simulink model "HW1_9723052"  (R2020b)
settings: Solver=VariableStepAuto  StartTime=0.0  StopTime=45  RelTol=1e-3
InitFcn:
  | run('Transmitter.m')
StopFcn:
  | RxStream = out.RxStream
  | run('Receiver.m')
  | MY = out.MY
values from neighbouring files (symbols this model uses):
  alpha = 0.2    [Transmitter.m]
  Frame = reshape(Frames.',[1,R_a*C_a])    [Transmitter.m]
  H = [ 0,1,1,1,0,1,0,0,1,1,1,0,1,1,0,0,1,1,0,0,0,0,1,1,1,0,0,1,1,1,0,1,1,0,0,0,1,1,0,1,0,       1,0,0,1,0,0,0,0,1,1,0,0,1,1,0,0,0,0,0,1,0,1,0,0,1,1,1,0,0,0,0,1,1,0,1,1,0,1,1,1,1,       1,1,1,1,0,0,1,0,1,0,0,0,0,0,0,0,1,0,0,0,1,1,0,1,1,1,0,1,1,1,0,1,0,1,0,1,0,0,1,1,1,       0,1,0,1,0 ]    [Transmitter.m]
  hd = h(2:end).*conj(h(1:end-1))    [Transmitter.m]
  M = 16    [Transmitter.m]
  Rs = 10e3    (= 10000)    [Transmitter.m]
  span = 20    [Transmitter.m]
  SPS = 8    [Transmitter.m]
undefined symbols (not defined in the file or in its folder): magnitude, pskmod
libraries: simulink x6, commdigbbndpm3 x5, commdigbbndam3 x4, dspstat3 x2, commfilt2 x2, commchan3 x1, dspsrcs4 x1
settings Model: Creator=win_10  LastModifiedBy=bpc

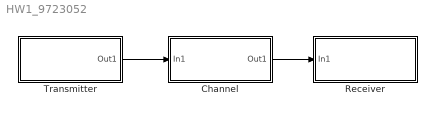
== system HW1_9723052 ==
  Channel : Subsystem
  Receiver : Subsystem
  Transmitter : Subsystem
  wires:
  Transmitter/1(Out1) -> Channel/1(In1)
  Channel/1(Out1) -> Receiver/1(In1)

== system HW1_9723052/Channel ==
  In1 : Inport
  AWGN Channel : commchan3/AWGN Channel  Commented=through  InputProcessing=Columns as channels (frame based)  seed=67  noiseMode="Signal to noise ratio  (Es/No)"  EbNodB=50  EsNodB=15  SNRdB=10  bitsPerSym=log2(M)  Ps=1/SPS  Tsym=1/Rs  variance=1
  Gain : Gain
  Out1 : Outport
  wires:
  In1/1 -> AWGN Channel/1
  AWGN Channel/1 -> Gain/1
  Gain/1 -> Out1/1

== system HW1_9723052/Receiver ==
  In1 : Inport
  Data Aided : Subsystem
  Downsample : DownSample  N=SPS  RateOptions=Allow multirate processing
  M&M : Subsystem  Commented=through
  Raised Cosine Receive Filter : commfilt2/Raised Cosine Receive Filter  filtType=Square root  R=alpha  filtSpan=span  N=SPS  downFactor=1  downOffset=0  filterGain=1  InputProcessing=Columns as channels (frame based)  RateOptions=Allow multirate processing  framing=Mute  checkCoeff=off  variableName=rcRxFilt  currentFiltSpan=span  D=(span)/2  inputOffset=0  sampMode=Mute  saveAsFlag=0  rateMode=Downsampling  checkGain=Normalized  launchFVT=on  roundingMode=Floor  overflowMode=off  coeffDataTypeStr=Inherit: Same word length as input  coeffMin=[]  coeffMax=[]  coeffLastDataTypeStr=Inherit: Same word length as input  accumDataTypeStr=Inherit: Same as product output  accumLastDataTypeStr=Inherit: Same as product output  outputDataTypeStr=Inherit: Same as accumulator  outputMin=[]  outputMax=[]  outputLastDataTypeStr=Inherit: Same as accumulator
      settings: SourceProductName=Communications Toolbox
  wires:
  In1/1 -> Raised Cosine Receive Filter/1
  Raised Cosine Receive Filter/1 -> Downsample/1
  Downsample/1 -> M&M/1(In1), Data Aided/1(Input)

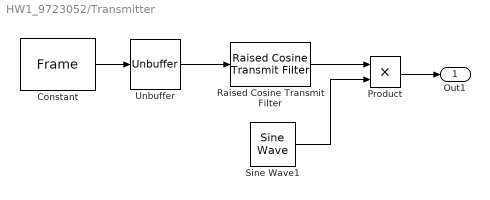
== system HW1_9723052/Transmitter ==
  Constant : Constant  Value=Frame  SampleTime=(length(Frame))/Rs
  Product : Product
  Raised Cosine Transmit Filter : commfilt2/Raised Cosine Transmit Filter  filtType=Square root  R=alpha  filtSpan=span  N=SPS  filterGain=1  InputProcessing=Columns as channels (frame based)  RateOptions=Allow multirate processing  framing=Mute  checkCoeff=off  variableName=rcTxFilt  checkGain=Normalized  sampMode=Mute  saveAsFlag=0  currentFiltSpan=span  D=(span)/2  launchFVT=on  roundingMode=Floor  overflowMode=off  coeffDataTypeStr=Inherit: Same word length as input  coeffMin=[]  coeffMax=[]  coeffLastDataTypeStr=Inherit: Same word length as input  outputDataTypeStr=Inherit: Same as accumulator  outputMin=[]  outputMax=[]  outputLastDataTypeStr=Inherit: Same as accumulator
      settings: SourceProductName=Communications Toolbox
  Sine Wave1 : dspsrcs4/Sine Wave  Amplitude=1  Frequency=(0.0001*Rs)  Phase=0  SampleMode=Discrete  OutComplex=Complex  CompMethod=Trigonometric fcn  TableSize=Speed  SampleTime=1/(SPS*Rs)  SamplesPerFrame=1  ResetState=Restart at time zero  OutputFrames=off  dataType=double  wordLen=16  udDataType=sfix(16)  fracBitsMode=Best precision  numFracBits=15  OutDataTypeStr=double  LastOutDataTypeStr=double
  Unbuffer : Unbuffer
  Out1 : Outport
  wires:
  Constant/1 -> Unbuffer/1
  Unbuffer/1 -> Raised Cosine Transmit Filter/1
  Sine Wave1/1 -> Product/2
  Raised Cosine Transmit Filter/1 -> Product/1
  Product/1 -> Out1/1

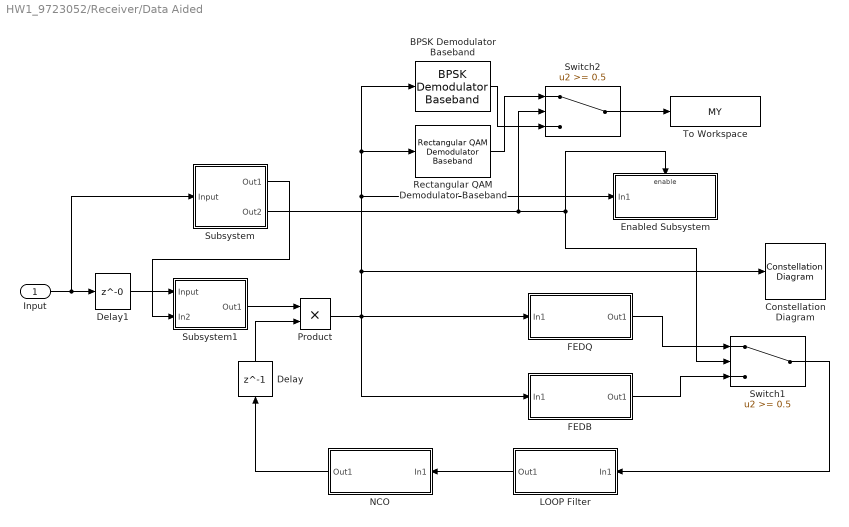
== system HW1_9723052/Receiver/Data Aided ==
  Input : Inport
  BPSK Demodulator Baseband : commdigbbndpm3/BPSK Demodulator Baseband  DecType=Hard decision  VarSource=Dialog  Variance=1  Ph=0  outDtype=Inherit via internal rule  derotateFactorWordLen=16  derotateFactorDataTypeStr=Inherit: Same word length as input  derotateFactorLastDataTypeStr=Inherit: Same word length as input
      settings: SourceProductName=Communications Toolbox
  Constellation Diagram : ConstellationDiagram
  Delay : Delay  DelayLength=1
  Delay1 : Delay  DelayLength=0
  Enabled Subsystem : Subsystem  TreatAsAtomicUnit=on
  FEDB : Subsystem
  FEDQ : Subsystem
  LOOP Filter : Subsystem
  NCO : Subsystem
  Product : Product
  Rectangular QAM Demodulator Baseband : commdigbbndam3/Rectangular QAM Demodulator Baseband  M=M  OutType=Integer  DecType=Hard decision  VarSource=Dialog  Variance=1  Dec=Gray  Mapping=[0:15]  PowType=Min. distance between symbols  MinDist=2  AvgPow=1  PeakPow=1  Ph=0  outDtype1=Inherit via internal rule  outDtype2=Inherit via internal rule  derotateFactorWordLen=16  derotateFactorDataTypeStr=Inherit: Same word length as input  derotateFactorLastDataTypeStr=Inherit: Same word length as input  denormFactorWordLen=16  denormFactorDataTypeStr=Inherit: Same word length as input  denormFactorLastDataTypeStr=Inherit: Same word length as input  prodOutWordLen=32  prodOutOverflowMode=Wrap  prodOutRoundingMode=Floor  prodOutOvFlMode=off  prodOutOvFlModeLastStrValue=off  sumWordLen=32
      settings: SourceProductName=Communications Toolbox
  Subsystem : Subsystem
  Subsystem1 : Subsystem
  Switch1 : Switch  Threshold=0.5
  Switch2 : Switch  Threshold=0.5
  To Workspace : ToWorkspace  VariableName=MY  SampleTime=-1
      settings: Save2DSignal=2-D array (concatenate along first dimension)
  wires:
  Delay/1 -> Product/2
  LOOP Filter/1(Out1) -> NCO/1(In1)
  NCO/1(Out1) -> Delay/1
  Switch1/1 -> LOOP Filter/1(In1)
  FEDQ/1(Out1) -> Switch1/1
  FEDB/1(Out1) -> Switch1/3
  Input/1 -> Delay1/1, Subsystem/1(Input)
  Product/1 -> Rectangular QAM Demodulator Baseband/1, BPSK Demodulator Baseband/1, Enabled Subsystem/1(In1), Constellation Diagram/1, FEDB/1(In1), FEDQ/1(In1)
  Subsystem/1(Out1) -> Subsystem1/2(In2)
  Delay1/1 -> Subsystem1/1(Input)
  Subsystem1/1(Out1) -> Product/1
  Subsystem/2(Out2) -> Switch2/2, Enabled Subsystem/Enable, Switch1/2
  Rectangular QAM Demodulator Baseband/1 -> Switch2/1
  BPSK Demodulator Baseband/1 -> Switch2/3
  Switch2/1 -> To Workspace/1

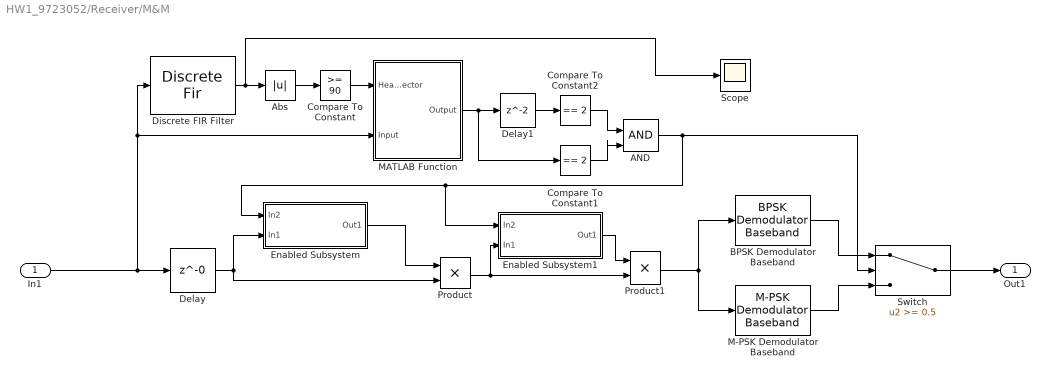
== system HW1_9723052/Receiver/M&M ==
  In1 : Inport
  AND : Logic  IconShape=distinctive  AllPortsSameDT=off  OutDataTypeStr=boolean
  Abs : Abs
  BPSK Demodulator Baseband : commdigbbndpm3/BPSK Demodulator Baseband  DecType=Hard decision  VarSource=Dialog  Variance=1  Ph=pi/M-pi/M*(M==2)  outDtype=Inherit via internal rule  derotateFactorWordLen=16  derotateFactorDataTypeStr=Inherit: Same word length as input  derotateFactorLastDataTypeStr=Inherit: Same word length as input
      settings: SourceProductName=Communications Toolbox
  Compare To Constant : simulink/Logic and Bit Operations/Compare To Constant  relop=>=  const=90  OutDataTypeStr=boolean
  Compare To Constant1 : simulink/Logic and Bit Operations/Compare To Constant  relop===  const=2  OutDataTypeStr=boolean
  Compare To Constant2 : simulink/Logic and Bit Operations/Compare To Constant  relop===  const=2  OutDataTypeStr=boolean
  Delay : Delay  DelayLength=0
  Delay1 : Delay  InputProcessing=Columns as channels (frame based)
  Discrete FIR Filter : DiscreteFir  Coefficients=fliplr(pskmod(H,2))
  Enabled Subsystem : Subsystem  TreatAsAtomicUnit=on
  Enabled Subsystem1 : Subsystem  TreatAsAtomicUnit=on
  M-PSK Demodulator Baseband : commdigbbndpm3/M-PSK Demodulator Baseband  M=M  OutType=Integer  DecType=Hard decision  VarSource=Dialog  Variance=1  Dec=Gray  Mapping=[0:7]  Ph=pi/M-pi/M*(M==2)  outDtype1=Inherit via internal rule  outDtype2=Inherit via internal rule  derotateFactorWordLen=16  derotateFactorDataTypeStr=Inherit: Same word length as input  derotateFactorLastDataTypeStr=Inherit: Same word length as input
      settings: SourceProductName=Communications Toolbox
  MATLAB Function : MATLAB Function  TreatAsAtomicUnit=on
  Product : Product
  Product1 : Product
  Scope : Scope
  Switch : Switch  Threshold=0.5
  Out1 : Outport
  wires:
  AND/1 -> Switch/2, Enabled Subsystem/1(In2), Enabled Subsystem1/1(In2)
  In1/1 -> Delay/1, MATLAB Function/2(Input), Discrete FIR Filter/1
  MATLAB Function/1(Output) -> Compare To Constant1/1, Delay1/1
  Compare To Constant/1 -> MATLAB Function/1(Header_Detector)
  Delay/1 -> Enabled Subsystem/2(In1), Product/2
  Discrete FIR Filter/1 -> Scope/1, Abs/1
  Abs/1 -> Compare To Constant/1
  Delay1/1 -> Compare To Constant2/1
  Compare To Constant1/1 -> AND/2
  Enabled Subsystem1/1(Out1) -> Product1/1
  Product/1 -> Product1/2, Enabled Subsystem1/2(In1)
  Enabled Subsystem/1(Out1) -> Product/1
  Compare To Constant2/1 -> AND/1
  Switch/1 -> Out1/1
  Product1/1 -> M-PSK Demodulator Baseband/1, BPSK Demodulator Baseband/1
  M-PSK Demodulator Baseband/1 -> Switch/3
  BPSK Demodulator Baseband/1 -> Switch/1

== system HW1_9723052/Receiver/Data Aided/Enabled Subsystem ==
  In1 : Inport
  Enable : EnablePort
  Rectangular QAM Demodulator Baseband : commdigbbndam3/Rectangular QAM Demodulator Baseband  M=M  OutType=Integer  DecType=Hard decision  VarSource=Dialog  Variance=1  Dec=Gray  Mapping=[0:15]  PowType=Min. distance between symbols  MinDist=2  AvgPow=1  PeakPow=1  Ph=0  outDtype1=Inherit via internal rule  outDtype2=Inherit via internal rule  derotateFactorWordLen=16  derotateFactorDataTypeStr=Inherit: Same word length as input  derotateFactorLastDataTypeStr=Inherit: Same word length as input  denormFactorWordLen=16  denormFactorDataTypeStr=Inherit: Same word length as input  denormFactorLastDataTypeStr=Inherit: Same word length as input  prodOutWordLen=32  prodOutOverflowMode=Wrap  prodOutRoundingMode=Floor  prodOutOvFlMode=off  prodOutOvFlModeLastStrValue=off  sumWordLen=32
      settings: SourceProductName=Communications Toolbox
  To Workspace : ToWorkspace  VariableName=RxStream  SampleTime=-1
      settings: Save2DSignal=2-D array (concatenate along first dimension)
  wires:
  Rectangular QAM Demodulator Baseband/1 -> To Workspace/1
  In1/1 -> Rectangular QAM Demodulator Baseband/1

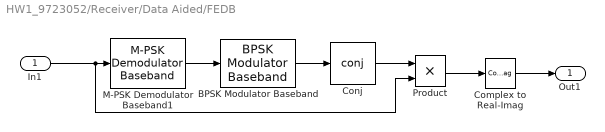
== system HW1_9723052/Receiver/Data Aided/FEDB ==
  In1 : Inport
  BPSK Modulator Baseband : commdigbbndpm3/BPSK Modulator Baseband  Ph=0  outDtype=double  outWordLen=16  outUDDataType=sfix(16)  outFracLenMode=Best precision  outFracLen=15  outDataTypeStr=double  outLastDataTypeStr=double
      settings: SourceProductName=Communications Toolbox
  Complex to Real-Imag : ComplexToRealImag  Output=Imag
  Conj : Math  Operator=conj  SaturateOnIntegerOverflow=on
  M-PSK Demodulator Baseband1 : commdigbbndpm3/M-PSK Demodulator Baseband  M=2  OutType=Integer  DecType=Hard decision  VarSource=Dialog  Variance=1  Dec=Gray  Mapping=[0:7]  Ph=0  outDtype1=Inherit via internal rule  outDtype2=Inherit via internal rule  derotateFactorWordLen=16  derotateFactorDataTypeStr=Inherit: Same word length as input  derotateFactorLastDataTypeStr=Inherit: Same word length as input
  Product : Product
  Out1 : Outport
  wires:
  In1/1 -> M-PSK Demodulator Baseband1/1, Product/2
  M-PSK Demodulator Baseband1/1 -> BPSK Modulator Baseband/1
  BPSK Modulator Baseband/1 -> Conj/1
  Conj/1 -> Product/1
  Complex to Real-Imag/1 -> Out1/1
  Product/1 -> Complex to Real-Imag/1

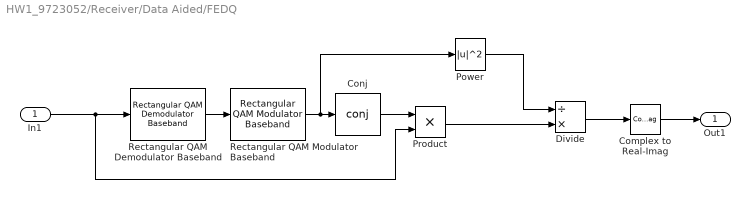
== system HW1_9723052/Receiver/Data Aided/FEDQ ==
  In1 : Inport
  Complex to Real-Imag : ComplexToRealImag  Output=Imag
  Conj : Math  Operator=conj  SaturateOnIntegerOverflow=on
  Divide : Product  Inputs=/*
  Power : Math  Operator=magnitude^2  SaturateOnIntegerOverflow=on
  Product : Product
  Rectangular QAM Demodulator Baseband : commdigbbndam3/Rectangular QAM Demodulator Baseband  M=M  OutType=Integer  DecType=Hard decision  VarSource=Dialog  Variance=1  Dec=Gray  Mapping=[0:15]  PowType=Min. distance between symbols  MinDist=2  AvgPow=1  PeakPow=1  Ph=0  outDtype1=Inherit via internal rule  outDtype2=Inherit via internal rule  derotateFactorWordLen=16  derotateFactorDataTypeStr=Inherit: Same word length as input  derotateFactorLastDataTypeStr=Inherit: Same word length as input  denormFactorWordLen=16  denormFactorDataTypeStr=Inherit: Same word length as input  denormFactorLastDataTypeStr=Inherit: Same word length as input  prodOutWordLen=32  prodOutOverflowMode=Wrap  prodOutRoundingMode=Floor  prodOutOvFlMode=off  prodOutOvFlModeLastStrValue=off  sumWordLen=32
      settings: SourceProductName=Communications Toolbox
  Rectangular QAM Modulator Baseband : commdigbbndam3/Rectangular QAM Modulator Baseband  M=M  InType=Integer  Enc=Gray  Mapping=[0:15]  PowType=Min. distance between symbols  MinDist=2  AvgPow=1  PeakPow=1  Ph=0  outDtype=double  outWordLen=16  outUDDataType=sfix(16)  outFracLenMode=Best precision  outFracLen=15  outDataTypeStr=double  outLastDataTypeStr=double
      settings: SourceProductName=Communications Toolbox
  Out1 : Outport
  wires:
  In1/1 -> Rectangular QAM Demodulator Baseband/1, Product/2
  Conj/1 -> Product/1
  Complex to Real-Imag/1 -> Out1/1
  Rectangular QAM Demodulator Baseband/1 -> Rectangular QAM Modulator Baseband/1
  Rectangular QAM Modulator Baseband/1 -> Power/1, Conj/1
  Divide/1 -> Complex to Real-Imag/1
  Power/1 -> Divide/1
  Product/1 -> Divide/2

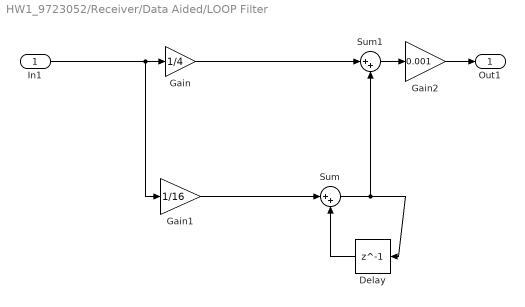
== system HW1_9723052/Receiver/Data Aided/LOOP Filter ==
  In1 : Inport
  Delay : Delay  DelayLength=1
  Gain : Gain  Gain=1/4
  Gain1 : Gain  Gain=1/16
  Gain2 : Gain  Gain=0.001
  Sum : Sum  Inputs=|++
  Sum1 : Sum  Inputs=|++
  Out1 : Outport
  wires:
  In1/1 -> Gain1/1, Gain/1
  Gain1/1 -> Sum/1
  Delay/1 -> Sum/2
  Sum/1 -> Sum1/2, Delay/1
  Gain/1 -> Sum1/1
  Sum1/1 -> Gain2/1
  Gain2/1 -> Out1/1

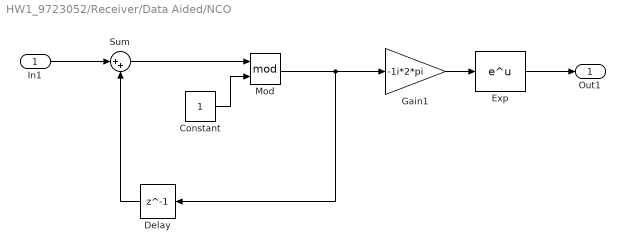
== system HW1_9723052/Receiver/Data Aided/NCO ==
  In1 : Inport
  Constant : Constant
  Delay : Delay  DelayLength=1
  Exp : Math  SaturateOnIntegerOverflow=on
  Gain1 : Gain  Gain=-1i*2*pi
  Mod : Math  Operator=mod  SaturateOnIntegerOverflow=on
  Sum : Sum  Inputs=|++
  Out1 : Outport
  wires:
  Sum/1 -> Mod/1
  Constant/1 -> Mod/2
  Delay/1 -> Sum/2
  In1/1 -> Sum/1
  Mod/1 -> Delay/1, Gain1/1
  Gain1/1 -> Exp/1
  Exp/1 -> Out1/1

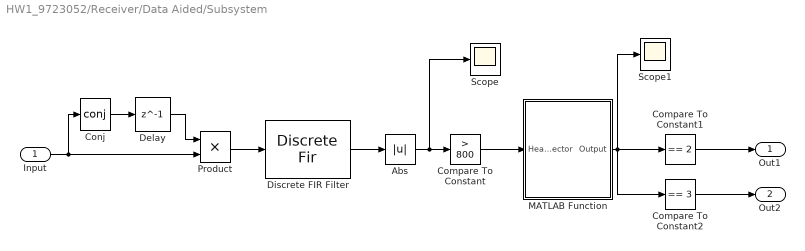
== system HW1_9723052/Receiver/Data Aided/Subsystem ==
  Input : Inport
  Abs : Abs
  Compare To Constant : simulink/Logic and Bit Operations/Compare To Constant  relop=>  const=800  OutDataTypeStr=boolean
  Compare To Constant1 : simulink/Logic and Bit Operations/Compare To Constant  relop===  const=2  OutDataTypeStr=boolean
  Compare To Constant2 : simulink/Logic and Bit Operations/Compare To Constant  relop===  const=3  OutDataTypeStr=boolean
  Conj : Math  Operator=conj  SaturateOnIntegerOverflow=on
  Delay : Delay  DelayLength=1
  Discrete FIR Filter : DiscreteFir  Coefficients=fliplr(hd)
  MATLAB Function : MATLAB Function  TreatAsAtomicUnit=on
  Product : Product
  Scope : Scope
  Scope1 : Scope
  Out1 : Outport
  Out2 : Outport  Port=2
  wires:
  Compare To Constant1/1 -> Out1/1
  MATLAB Function/1(Output) -> Compare To Constant2/1, Scope1/1, Compare To Constant1/1
  Compare To Constant/1 -> MATLAB Function/1(Header_Detector)
  Discrete FIR Filter/1 -> Abs/1
  Compare To Constant2/1 -> Out2/1
  Abs/1 -> Scope/1, Compare To Constant/1
  Input/1 -> Conj/1, Product/2
  Product/1 -> Discrete FIR Filter/1
  Conj/1 -> Delay/1
  Delay/1 -> Product/1

== system HW1_9723052/Receiver/Data Aided/Subsystem1 ==
  Input : Inport
  In2 : Inport  Port=2
  Delay : Delay  DelayLength=1
  Product : Product
  Subsystem : Subsystem
  Out1 : Outport
  wires:
  In2/1 -> Subsystem/Enable
  Product/1 -> Subsystem/1(In1), Out1/1
  Input/1 -> Product/2
  Subsystem/1(Out1) -> Delay/1
  Delay/1 -> Product/1

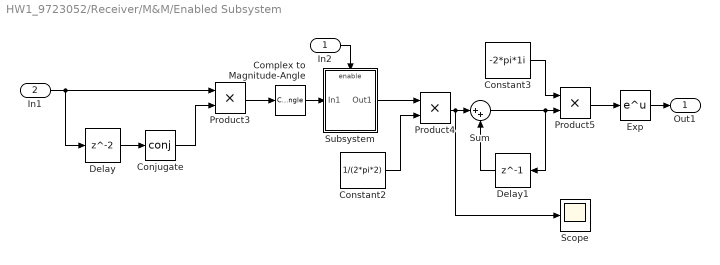
== system HW1_9723052/Receiver/M&M/Enabled Subsystem ==
  In2 : Inport
  In1 : Inport  Port=2
  Complex to Magnitude-Angle : ComplexToMagnitudeAngle  Output=Angle
  Conjugate : Math  Operator=conj  SignedPower=on  RndMeth=Zero  SaturateOnIntegerOverflow=on
  Constant2 : Constant  Value=1/(2*pi*2)
  Constant3 : Constant  Value=-2*pi*1i
  Delay : Delay
  Delay1 : Delay  DelayLength=1
  Exp : Math  SaturateOnIntegerOverflow=on
  Product3 : Product
  Product4 : Product
  Product5 : Product
  Scope : Scope
  Subsystem : Subsystem
  Sum : Sum  Inputs=|++
  Out1 : Outport
  wires:
  In1/1 -> Product3/1, Delay/1
  Delay/1 -> Conjugate/1
  Conjugate/1 -> Product3/2
  Product3/1 -> Complex to Magnitude-Angle/1
  Constant2/1 -> Product4/2
  Product5/1 -> Exp/1
  Constant3/1 -> Product5/1
  Exp/1 -> Out1/1
  In2/1 -> Subsystem/Enable
  Complex to Magnitude-Angle/1 -> Subsystem/1(In1)
  Subsystem/1(Out1) -> Product4/1
  Product4/1 -> Scope/1, Sum/1
  Sum/1 -> Delay1/1, Product5/2
  Delay1/1 -> Sum/2

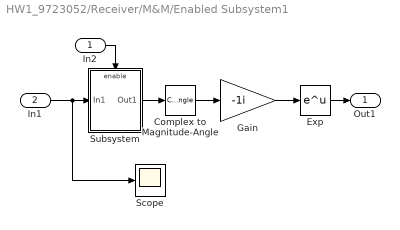
== system HW1_9723052/Receiver/M&M/Enabled Subsystem1 ==
  In2 : Inport
  In1 : Inport  Port=2
  Complex to Magnitude-Angle : ComplexToMagnitudeAngle  Output=Angle
  Exp : Math  SaturateOnIntegerOverflow=on
  Gain : Gain  Gain=-1i
  Scope : Scope
  Subsystem : Subsystem
  Out1 : Outport
  wires:
  Gain/1 -> Exp/1
  Exp/1 -> Out1/1
  In2/1 -> Subsystem/Enable
  In1/1 -> Scope/1, Subsystem/1(In1)
  Subsystem/1(Out1) -> Complex to Magnitude-Angle/1
  Complex to Magnitude-Angle/1 -> Gain/1

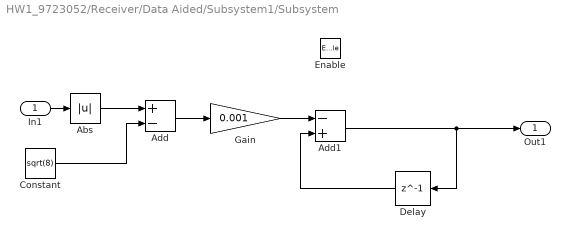
== system HW1_9723052/Receiver/Data Aided/Subsystem1/Subsystem ==
  In1 : Inport
  Enable : EnablePort
  Abs : Abs
  Add : Sum  Inputs=+-
  Add1 : Sum  Inputs=-+
  Constant : Constant  Value=sqrt(8)
  Delay : Delay  DelayLength=1
  Gain : Gain  Gain=0.001
  Out1 : Outport
  wires:
  Constant/1 -> Add/2
  In1/1 -> Abs/1
  Add/1 -> Gain/1
  Gain/1 -> Add1/1
  Delay/1 -> Add1/2
  Add1/1 -> Delay/1, Out1/1
  Abs/1 -> Add/1

== system HW1_9723052/Receiver/M&M/Enabled Subsystem/Subsystem ==
  In1 : Inport
  Enable : EnablePort
  Moving Average : dspstat3/Moving Average  Method=Sliding window  ForgettingFactorPort=off  SpecifyWindowLength=on  WindowLength=8  ForgettingFactor=0.9  SimulateUsing=Code generation
  Out1 : Outport
  wires:
  In1/1 -> Moving Average/1
  Moving Average/1 -> Out1/1

== system HW1_9723052/Receiver/M&M/Enabled Subsystem1/Subsystem ==
  In1 : Inport
  Enable : EnablePort
  Moving Average : dspstat3/Moving Average  Method=Sliding window  ForgettingFactorPort=off  SpecifyWindowLength=on  WindowLength=8  ForgettingFactor=0.9  SimulateUsing=Code generation
  Out1 : Outport
  wires:
  In1/1 -> Moving Average/1
  Moving Average/1 -> Out1/1

== matlab function HW1_9723052/Receiver/Data Aided/Subsystem/MATLAB Function ==
  data: Header_Detector input; Output output
function Output = Frame_Detector( Header_Detector )
    
    persistent N1 ;
    persistent Z1 ;
    persistent i1 ;
    persistent i2 ;
    persistent D ;
    
    if isempty(N1) && isempty(Z1) && isempty(i1) && isempty(i2)
        N1 = 0 ;
        Z1 = 0 ;
        i1 = 0 ;
        i2 = 0 ;
        D  = 1 ;
    end
    
    Delay = 1 ;
    Delay_Value = 1 ;
    Header_Detected_Value = 1 ;
    Header_Value = 1 ;
    Pilot_Value = 2 ;
    Data_Value = 3 ;
    Data_Part = 3 ;
    Zero_Part = 2 ;
    N = 256 ;
    Z = 10 ;
    
    if Header_Detector == 1
        K = Header_Detected_Value ;
        N1 = 1 ;  
        Z1 = 1 ;
        i1 = 0 ;
        i2 = 0 ;
    elseif ( i1 + i2 ) == ( Data_Part + Zero_Part )
        K = Header_Value ; 
    elseif N1 == (N + 1)
        K = Pilot_Value ;
        Z1 = Z1 + 1 ;
        if Z1 == (Z + 1)
           i2 = i2 + 1 ;
        end
    elseif N1 >= 1 && N1 <= N
        K = Data_Value ;
        N1 = N1 + 1 ;
        if N1 == (N + 1)
           i1 = i1 + 1 ;
        end
    elseif D >= 1 && D <= Delay
        K = Delay_Value ;
        D = D + 1 ;
    else
        K = Header_Value ;
    end

    if N1 == (N + 1) && Z1 == (Z + 1)
       N1 = 1 ;
       Z1 = 1 ;
    end
    
    Output = K ;

end



% function y = fcn(En)
% L = 916;
% persistent count
% if isempty(count)
%     count = 0;
% end
% 
% if En == 1
%     count = 0;
% else
%     count = count + 1;
% end
% 
% if (count <= 128 && count >=1)
%     y = 1; %preamble
% elseif ((count > 384 && count <= 394) ||(count > 650 && count <= 660))
%     y= 2; %pilot
% else
%     y = 3; %data
% end
% end

== matlab function HW1_9723052/Receiver/M&M/MATLAB Function ==
  data: Header_Detector input; Output output; Input input
function Output = Frame_Detector( Header_Detector , Input )
    
    persistent N1 ;
    persistent Z1 ;
    persistent i1 ;
    persistent i2 ;
    persistent D ;
    
    if isempty(N1) && isempty(Z1) && isempty(i1) && isempty(i2)
        N1 = 0 ;
        Z1 = 0 ;
        i1 = 0 ;
        i2 = 0 ;
        D  = 1 ;
    end
    
    Delay = 20 ;
    Delay_Value = 0 ;
    Header_Detected_Value = 5 ;
    Header_Value = 1 ;
    Zero_Value = 2 ;
    Data_Part = 3 ;
    Zero_Part = 2 ;
    N = 256 ;
    Z = 10 ;
    
    if Header_Detector == 1
        K = Header_Detected_Value ;
        N1 = 1 ;  
        Z1 = 1 ;
        i1 = 0 ;
        i2 = 0 ;
    elseif ( i1 + i2 ) == ( Data_Part + Zero_Part )
        K = Header_Value ; 
    elseif N1 == (N + 1)
        K = Zero_Value ;
        Z1 = Z1 + 1 ;
        if Z1 == (Z + 1)
           i2 = i2 + 1 ;
        end
    elseif N1 >= 1 && N1 <= N
        K = Input ;
        N1 = N1 + 1 ;
        if N1 == (N + 1)
           i1 = i1 + 1 ;
        end
    elseif D >= 1 && D <= Delay
        K = Delay_Value ;
        D = D + 1 ;
    else
        K = Header_Value ;
    end

    if N1 == (N + 1) && Z1 == (Z + 1)
       N1 = 1 ;
       Z1 = 1 ;
    end
    
    Output = K ;

end
